simulink model "Simulink_Interferencia"  (R2021b)
settings: Solver=VariableStepAuto  StartTime=0.0  StopTime=Inf  RelTol=1e-3
libraries: commanabbnd3 x2, dspsnks4 x1, dspsrcs4 x1, dspvision x1
settings Model: Creator=enrique  LastModifiedBy=enrique

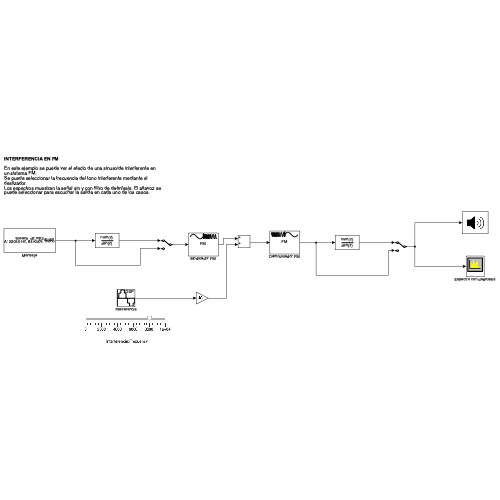
[thumbnail: Simulink's stored preview of the top-level diagram]
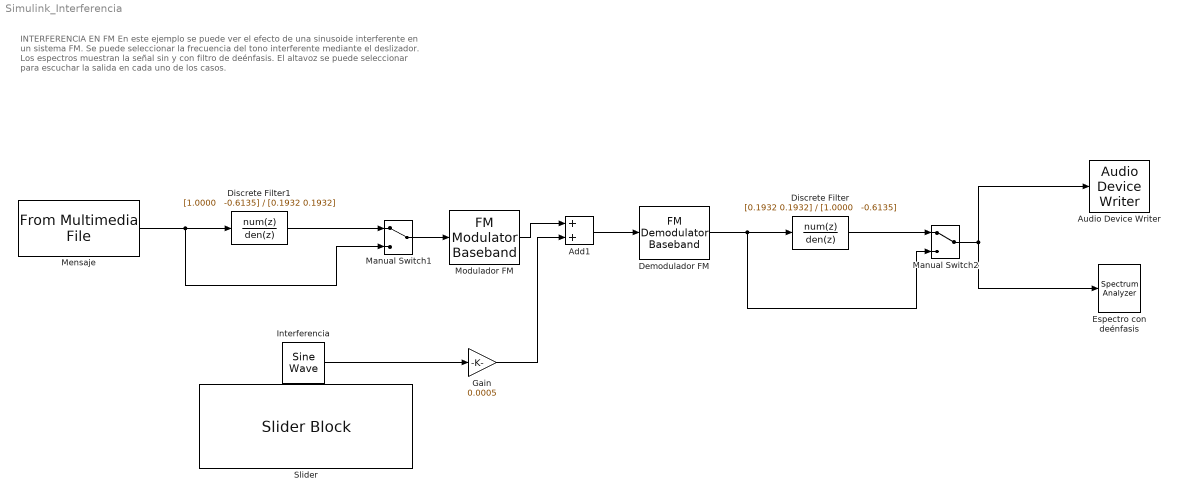
== system Simulink_Interferencia ==
  note: INTERFERENCIA EN FM
      |
      | En este ejemplo se puede ver el efecto de una sinusoide interferente en un sistema FM.
      | Se puede seleccionar la frecuencia del tono interferente mediante el deslizador.
      | Los espectros muestran la señal sin y con filtro de deénfasis. El altavoz se puede seleccionar para escuchar la salida en cada uno de los casos.
  Add1 : Sum
  Audio Device Writer : dspsnks4/Audio Device Writer  Driver=CoreAudio  Device=Default  InheritSampleRate=on  SampleRate=44100  BitDepth=16-bit integer  BufferSize=4096  NumBuffers=10  DefaultOutputChannelMapping=on  OutputChannelMapping=1:2  OutputNumUnderrunSamples=off  DriverIdx=5  DeviceWarnFlag=''
  Demodulador FM : commanabbnd3/FM Demodulator Baseband   FrequencyDeviation=75  SimulateUsing=Code generation
      settings: SourceProductBaseCode=CM
  Discrete Filter : DiscreteFilter  Numerator=[0.1932 0.1932]  Denominator="[1.0000   -0.6135]"  InputProcessing=Columns as channels (frame based)
  Discrete Filter1 : DiscreteFilter  Numerator="[1.0000   -0.6135]"  Denominator=[0.1932 0.1932]  InputProcessing=Columns as channels (frame based)
  Espectro con deénfasis : SpectrumAnalyzer
  Gain : Gain  Gain=0.0005
  Interferencia : dspsrcs4/Sine Wave  Amplitude=1  Frequency=8022.388059701493  Phase=0  SampleMode=Discrete  OutComplex=Real  CompMethod=Trigonometric fcn  TableSize=Speed  SampleTime=1/22050  SamplesPerFrame=1024  ResetState=Restart at time zero  OutputFrames=off  dataType=double  wordLen=16  udDataType=sfix(16)  fracBitsMode=Best precision  numFracBits=15  OutDataTypeStr=double  LastOutDataTypeStr=double
  Manual Switch1 : ManualSwitch
  Manual Switch2 : ManualSwitch
  Mensaje : dspvision/From Multimedia File  inputFilename=speech_dft.mp3  readRange=[1 Inf]  loop=on  numPlays=inf  outputStreams=Audio only  videoDataType=single  audioDataType=double  inheritSampleTime=on  userDefinedSampleTime=1/30  noAudioOutput=off  isIntensityVideo=off  fourcc=RGB  colorVideoFormat=Separate color signals  outputEOF=off  dataOrg=Column-major  audioFrameSize=1024  computeAudioFrameSize=off  outSamplingMode=Sample based
  Modulador FM : commanabbnd3/FM Modulator Baseband  FrequencyDeviation=75  SimulateUsing=Code generation
      settings: SourceProductBaseCode=CM
  Slider : SliderBlock  LabelPosition=Bottom  ScaleMax=10000  TickInterval=2000
  wires:
  Interferencia/1 -> Gain/1
  Gain/1 -> Add1/2
  Modulador FM/1 -> Add1/1
  Add1/1 -> Demodulador FM/1
  Discrete Filter1/1 -> Manual Switch1/1
  Manual Switch1/1 -> Modulador FM/1
  Discrete Filter/1 -> Manual Switch2/1
  Manual Switch2/1 -> Audio Device Writer/1, Espectro con deénfasis/1
  Demodulador FM/1 -> Discrete Filter/1, Manual Switch2/2
  Mensaje/1 -> Manual Switch1/2, Discrete Filter1/1
